simulink model "HighSpeedOperation"  (R2023a)
settings: Solver=VariableStepAuto  StartTime=0.0  StopTime=12  MaxStep=.00001  RelTol=.00001
values from neighbouring files (symbols this model uses):
  B = .005752    (= 0.005752)    [parameters.m]
  Fs = 5000    [parameters.m]
  I_rated = P_rated/(sqrt(3)*VLL_rms*.9*.9)    [parameters.m]
  J = .02    (= 0.02)    [parameters.m]
  lambda_r_rated = 0.94    [parameters.m]
  Llr = .005974    (= 0.005974)    [parameters.m]
  Lls = .005974    (= 0.005974)    [parameters.m]
  Lm = .2037    (= 0.2037)    [parameters.m]
  Lr = Lm+Llr    (= 0.209674)    [parameters.m]
  Ls = Lm+Lls    (= 0.209674)    [parameters.m]
  P = 4    [parameters.m]
  Rs = 1.115    [parameters.m]
  sigma = 1-((Lm)^2)/(Lr*Ls)    (= 0.0561719130296)    [parameters.m]
  Tr = Lr/Rr    (= 0.193604801477)    [parameters.m]
  Vdc = 600    [parameters.m]
  Vs_max = Vdc/sqrt(3)    [parameters.m]
libraries: slpidlib x7, spsMosfetLib x6, spsabctoAlphaBetaZeroLib x4, spsCurrentMeasurementLib x2, simulink x2, SignalEditorBlockLib x2, spsAsynchronousMachineSIUnitsLib x1, spsDCVoltageSourceLib x1, sps_lib x1
(part 1 of 2)
settings Model: Creator=User  LastModifiedBy=User
settings DebuggingCC: IgnoredZcDiagnostic=none

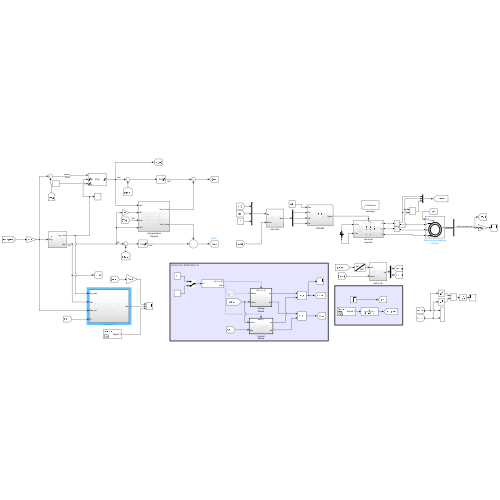
[thumbnail: Simulink's stored preview of the top-level diagram]
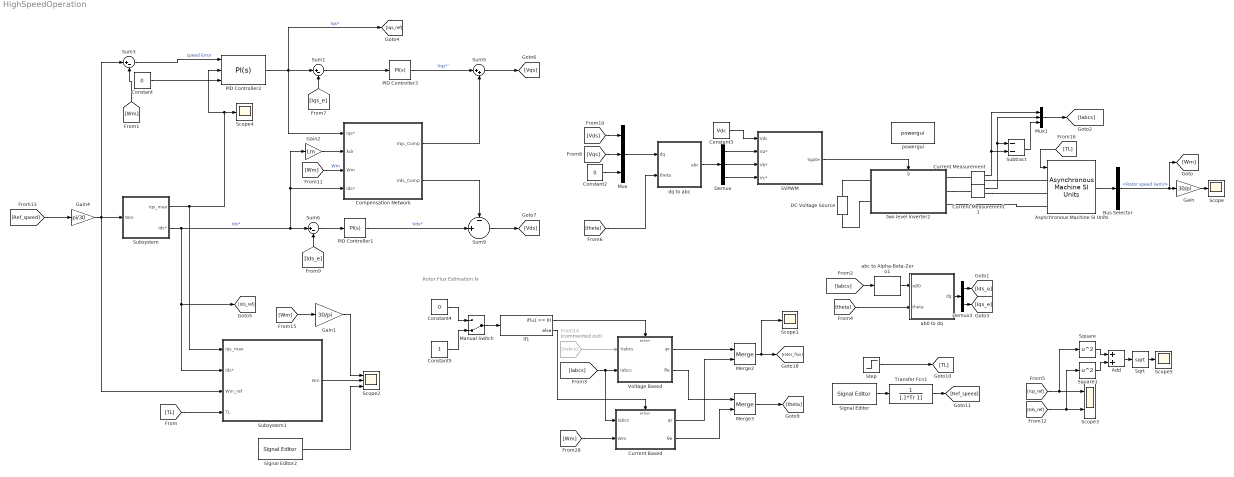
== system HighSpeedOperation ==
  note: Rotor Flux Estimation λr
  Add : Sum
  Asynchronous Machine SI Units : spsAsynchronousMachineSIUnitsLib/Asynchronous Machine SI Units  RotorType=Squirrel-cage  PresetModel="01:  5 HP   460 V 60Hz 1750 RPM"  MechanicalLoad=Torque Tm  ShowDetailedParameters=on  ReferenceFrame=Stationary  Units=SI  MeasurementBus=off  NominalParameters=[3730 460 60]  VoltageRatio=1  Stator=[1.115 0.005974]  Rotor=[1.083 0.005974]  Cage1=[0.4155 0.002066]  Cage2=[0.4168 0.0003495]  Lm=0.2037  Mechanical=[0.02 0.005752 2]  PolePairs=2  InitialConditions=[1 0 0 0 0 0 0 0]  SimulateSaturation=off  Saturation=[14.03593122, 27.81365428, 53.79336849, 72.68890987, 97.98006896, 148.6815601, 215.7428561, 302.9841135, 428.7778367 ; 230, 322, 414, 460, 506, 552, 598, 644, 690]  LoadFlowParameters=1492000  TsPowergui=0  TsBlock=-1  IterativeModel=Trapezoidal non iterative  IterativeDiscreteModel=Trapezoidal non iterative  Pmec=1.492e+006
  Bus Selector : BusSelector  OutputSignals=Mechanical.Rotor speed (wm)
  Compensation Network : Subsystem
  Constant : Constant  Value=0
  Constant2 : Constant  Value=0
  Constant3 : Constant  Value=Vdc
  Constant4 : Constant  Value=0
  Constant5 : Constant
  Current Based : Subsystem
  Current Measurement : spsCurrentMeasurementLib/Current Measurement  PhasorSimulation=off  OutputType=Complex  PSBequivalent=0
  Current Measurement1 : spsCurrentMeasurementLib/Current Measurement  PhasorSimulation=off  OutputType=Complex  PSBequivalent=0
  DC Voltage Source : spsDCVoltageSourceLib/DC Voltage Source  Amplitude=Vdc  Measurements=None
  Demux : Demux  Outputs=3
  Demux3 : Demux  Outputs=2
  From14 : From  Commented=on  GotoTag=Vabcs  TagVisibility=global
  Gain : Gain  Gain=30/pi
  Gain1 : Gain  Gain=30/pi
  Gain2 : Gain  Gain=Lm
  Gain4 : Gain  Gain=pi/30
  If1 : If  IfExpression=u1 == 0
  Manual Switch : ManualSwitch  CurrentSetting=0
  Merge2 : Merge
  Merge3 : Merge
  Mux : Mux  Inputs=3
  Mux1 : Mux  Inputs=3
  PID Controller1 : slpidlib/PID Controller  Controller=PI  Form=Parallel  TimeDomain=Continuous-time  UseExternalTs=off  SampleTime=-1  IntegratorMethod=Forward Euler  FilterMethod=Forward Euler  ControllerParametersSource=internal  P=8.96154169507065  I=1405.53236610577  UseKiTs=off  D=0  N=100  UseFilter=on  TunerSelectOption=Transfer Function Based (PID Tuner App)  InitialConditionSource=internal  InitialConditionForIntegrator=0  InitialConditionForFilter=0  DifferentiatorICPrevScaledInput=0  ExternalReset=none  TrackingMode=off  Kt=1  LimitOutput=on  SatLimitsSource=internal  UpperSaturationLimit=inf  LowerSaturationLimit=-inf  LinearizeAsGain=on  AntiWindupMode=clamping  Kb=1  LimitIntegrator=off  UpperIntegratorSaturationLimit=inf  LowerIntegratorSaturationLimit=-inf  POutMin=[]  POutMax=[]  IOutMin=[]  IOutMax=[]  DOutMin=[]  DOutMax=[]  NOutMin=[]  NOutMax=[]  SumOutMin=[]  SumOutMax=[]  SaturationOutMin=[]  SaturationOutMax=[]  PParamMin=[]  PParamMax=[]  IParamMin=[]  IParamMax=[]  DParamMin=[]  DParamMax=[]  NParamMin=[]  NParamMax=[]  KbParamMin=[]  KbParamMax=[]  KtParamMin=[]  KtParamMax=[]  KbOutMin=[]  KbOutMax=[]  KtOutMin=[]  KtOutMax=[]  IntegratorOutMin=[]  IntegratorOutMax=[]  FilterOutMin=[]  FilterOutMax=[]  SumI1OutMin=[]  SumI1OutMax=[]  SumI2OutMin=[]  SumI2OutMax=[]  SumI3OutMin=[]  SumI3OutMax=[]  SumI4OutMin=[]  SumI4OutMax=[]  SumDOutMin=[]  SumDOutMax=[]  DifferentiatorOutMin=[]  DifferentiatorOutMax=[]  FilterDiffOutCoefMin=[]  FilterDiffOutCoefMax=[]  ReciprocalOutMin=[]  ReciprocalOutMax=[]  SumDenOutMin=[]  SumDenOutMax=[]  SumNumOutMin=[]  SumNumOutMax=[]  DivideOutMin=[]  DivideOutMax=[]  UdiffTsProdOutMin=[]  UdiffTsProdOutMax=[]  NTsProdOutMin=[]  NTsProdOutMax=[]  UintegralTsProdOutMin=[]  UintegralTsProdOutMax=[]  UngainTsProdOutMin=[]  UngainTsProdOutMax=[]  ClampingZeroOutDataTypeStr=Inherit: Inherit via back propagation  ClampingZeroOutMin=[]  ClampingZeroOutMax=[]  FilterDenConstantOutDataTypeStr=Inherit: Inherit via back propagation  FilterDenConstantOutMin=[]  FilterDenConstantOutMax=[]  PCopyOutDataTypeStr=Inherit: Inherit via back propagation  PCopyOutMin=[]  PCopyOutMax=[]  NCopyOutDataTypeStr=Inherit: Inherit via back propagation  NCopyOutMin=[]  NCopyOutMax=[]  IntegratorContinuousStateAttributes=''  IntegratorStateMustResolveToSignalObject=off  IntegratorRTWStateStorageClass=Auto  FilterContinuousStateAttributes=''  FilterStateMustResolveToSignalObject=off  FilterRTWStateStorageClass=Auto  ParallelPVariant=InternalParameters  IdealPVariant=Disabled  IVariant=InternalParameters  DVariant=Disabled  IntegratorVariant=Continuous  SatVariant=Enabled  AWVariant=ContClampingParallel  PCopyVariant=Disabled  TRVariant=Disabled  FdbkBlocksVariant=Forward  IdealPFdbkVariant=Disabled  SatFdbkVariant=Disabled  DerivativeFilterVariant=Disabled  NVariant=Disabled  NCopyVariant=Disabled_SignalSpec  FilterICVariant=Disabled  IntegratorICVariant=InternalICs  ExternalResetVariant=Disabled  TRSumVariant=Passthrough  SumFdbkVariant=Disabled  SumVariant=Sum_PI  TsampFilterVariant=InternalTs  TsampNgainVariant=Passthrough  TsampIntegralVariant=Disabled_SignalSpec  ExternalSaturationOutDataTypeStr=Inherit: Same as second input
  PID Controller2 : slpidlib/PID Controller  Controller=PI  Form=Parallel  TimeDomain=Continuous-time  UseExternalTs=off  SampleTime=-1  IntegratorMethod=Forward Euler  FilterMethod=Forward Euler  ControllerParametersSource=internal  P=3.31333209954479  I=19.3873586247509  UseKiTs=off  D=0  N=100  UseFilter=on  TunerSelectOption=Transfer Function Based (PID Tuner App)  InitialConditionSource=internal  InitialConditionForIntegrator=0  InitialConditionForFilter=0  DifferentiatorICPrevScaledInput=0  ExternalReset=none  TrackingMode=off  Kt=1  LimitOutput=on  SatLimitsSource=external  UpperSaturationLimit=inf  LowerSaturationLimit=-inf  LinearizeAsGain=on  AntiWindupMode=clamping  Kb=1  LimitIntegrator=off  UpperIntegratorSaturationLimit=inf  LowerIntegratorSaturationLimit=-inf  POutMin=[]  POutMax=[]  IOutMin=[]  IOutMax=[]  DOutMin=[]  DOutMax=[]  NOutMin=[]  NOutMax=[]  SumOutMin=[]  SumOutMax=[]  SaturationOutMin=[]  SaturationOutMax=[]  PParamMin=[]  PParamMax=[]  IParamMin=[]  IParamMax=[]  DParamMin=[]  DParamMax=[]  NParamMin=[]  NParamMax=[]  KbParamMin=[]  KbParamMax=[]  KtParamMin=[]  KtParamMax=[]  KbOutMin=[]  KbOutMax=[]  KtOutMin=[]  KtOutMax=[]  IntegratorOutMin=[]  IntegratorOutMax=[]  FilterOutMin=[]  FilterOutMax=[]  SumI1OutMin=[]  SumI1OutMax=[]  SumI2OutMin=[]  SumI2OutMax=[]  SumI3OutMin=[]  SumI3OutMax=[]  SumI4OutMin=[]  SumI4OutMax=[]  SumDOutMin=[]  SumDOutMax=[]  DifferentiatorOutMin=[]  DifferentiatorOutMax=[]  FilterDiffOutCoefMin=[]  FilterDiffOutCoefMax=[]  ReciprocalOutMin=[]  ReciprocalOutMax=[]  SumDenOutMin=[]  SumDenOutMax=[]  SumNumOutMin=[]  SumNumOutMax=[]  DivideOutMin=[]  DivideOutMax=[]  UdiffTsProdOutMin=[]  UdiffTsProdOutMax=[]  NTsProdOutMin=[]  NTsProdOutMax=[]  UintegralTsProdOutMin=[]  UintegralTsProdOutMax=[]  UngainTsProdOutMin=[]  UngainTsProdOutMax=[]  ClampingZeroOutDataTypeStr=Inherit: Inherit via back propagation  ClampingZeroOutMin=[]  ClampingZeroOutMax=[]  FilterDenConstantOutDataTypeStr=Inherit: Inherit via back propagation  FilterDenConstantOutMin=[]  FilterDenConstantOutMax=[]  PCopyOutDataTypeStr=Inherit: Inherit via back propagation  PCopyOutMin=[]  PCopyOutMax=[]  NCopyOutDataTypeStr=Inherit: Inherit via back propagation  NCopyOutMin=[]  NCopyOutMax=[]  IntegratorContinuousStateAttributes=''  IntegratorStateMustResolveToSignalObject=off  IntegratorRTWStateStorageClass=Auto  FilterContinuousStateAttributes=''  FilterStateMustResolveToSignalObject=off  FilterRTWStateStorageClass=Auto  ParallelPVariant=InternalParameters  IdealPVariant=Disabled  IVariant=InternalParameters  DVariant=Disabled  IntegratorVariant=Continuous  SatVariant=External  AWVariant=ContClampingParallel  PCopyVariant=Disabled  TRVariant=Disabled  FdbkBlocksVariant=Forward  IdealPFdbkVariant=Disabled  SatFdbkVariant=Disabled  DerivativeFilterVariant=Disabled  NVariant=Disabled  NCopyVariant=Disabled_SignalSpec  FilterICVariant=Disabled  IntegratorICVariant=InternalICs  ExternalResetVariant=Disabled  TRSumVariant=Passthrough  SumFdbkVariant=Disabled  SumVariant=Sum_PI  TsampFilterVariant=InternalTs  TsampNgainVariant=Passthrough  TsampIntegralVariant=Disabled_SignalSpec  ExternalSaturationOutDataTypeStr=Inherit: Same as second input
  PID Controller3 : slpidlib/PID Controller  Controller=PI  Form=Parallel  TimeDomain=Continuous-time  UseExternalTs=off  SampleTime=-1  IntegratorMethod=Forward Euler  FilterMethod=Forward Euler  ControllerParametersSource=internal  P=8.96154169507065  I=1405.53236610577  UseKiTs=off  D=0  N=100  UseFilter=on  TunerSelectOption=Transfer Function Based (PID Tuner App)  InitialConditionSource=internal  InitialConditionForIntegrator=0  InitialConditionForFilter=0  DifferentiatorICPrevScaledInput=0  ExternalReset=none  TrackingMode=off  Kt=1  LimitOutput=on  SatLimitsSource=internal  UpperSaturationLimit=inf  LowerSaturationLimit=-inf  LinearizeAsGain=on  AntiWindupMode=clamping  Kb=1  LimitIntegrator=off  UpperIntegratorSaturationLimit=inf  LowerIntegratorSaturationLimit=-inf  POutMin=[]  POutMax=[]  IOutMin=[]  IOutMax=[]  DOutMin=[]  DOutMax=[]  NOutMin=[]  NOutMax=[]  SumOutMin=[]  SumOutMax=[]  SaturationOutMin=[]  SaturationOutMax=[]  PParamMin=[]  PParamMax=[]  IParamMin=[]  IParamMax=[]  DParamMin=[]  DParamMax=[]  NParamMin=[]  NParamMax=[]  KbParamMin=[]  KbParamMax=[]  KtParamMin=[]  KtParamMax=[]  KbOutMin=[]  KbOutMax=[]  KtOutMin=[]  KtOutMax=[]  IntegratorOutMin=[]  IntegratorOutMax=[]  FilterOutMin=[]  FilterOutMax=[]  SumI1OutMin=[]  SumI1OutMax=[]  SumI2OutMin=[]  SumI2OutMax=[]  SumI3OutMin=[]  SumI3OutMax=[]  SumI4OutMin=[]  SumI4OutMax=[]  SumDOutMin=[]  SumDOutMax=[]  DifferentiatorOutMin=[]  DifferentiatorOutMax=[]  FilterDiffOutCoefMin=[]  FilterDiffOutCoefMax=[]  ReciprocalOutMin=[]  ReciprocalOutMax=[]  SumDenOutMin=[]  SumDenOutMax=[]  SumNumOutMin=[]  SumNumOutMax=[]  DivideOutMin=[]  DivideOutMax=[]  UdiffTsProdOutMin=[]  UdiffTsProdOutMax=[]  NTsProdOutMin=[]  NTsProdOutMax=[]  UintegralTsProdOutMin=[]  UintegralTsProdOutMax=[]  UngainTsProdOutMin=[]  UngainTsProdOutMax=[]  ClampingZeroOutDataTypeStr=Inherit: Inherit via back propagation  ClampingZeroOutMin=[]  ClampingZeroOutMax=[]  FilterDenConstantOutDataTypeStr=Inherit: Inherit via back propagation  FilterDenConstantOutMin=[]  FilterDenConstantOutMax=[]  PCopyOutDataTypeStr=Inherit: Inherit via back propagation  PCopyOutMin=[]  PCopyOutMax=[]  NCopyOutDataTypeStr=Inherit: Inherit via back propagation  NCopyOutMin=[]  NCopyOutMax=[]  IntegratorContinuousStateAttributes=''  IntegratorStateMustResolveToSignalObject=off  IntegratorRTWStateStorageClass=Auto  FilterContinuousStateAttributes=''  FilterStateMustResolveToSignalObject=off  FilterRTWStateStorageClass=Auto  ParallelPVariant=InternalParameters  IdealPVariant=Disabled  IVariant=InternalParameters  DVariant=Disabled  IntegratorVariant=Continuous  SatVariant=Enabled  AWVariant=ContClampingParallel  PCopyVariant=Disabled  TRVariant=Disabled  FdbkBlocksVariant=Forward  IdealPFdbkVariant=Disabled  SatFdbkVariant=Disabled  DerivativeFilterVariant=Disabled  NVariant=Disabled  NCopyVariant=Disabled_SignalSpec  FilterICVariant=Disabled  IntegratorICVariant=InternalICs  ExternalResetVariant=Disabled  TRSumVariant=Passthrough  SumFdbkVariant=Disabled  SumVariant=Sum_PI  TsampFilterVariant=InternalTs  TsampNgainVariant=Passthrough  TsampIntegralVariant=Disabled_SignalSpec  ExternalSaturationOutDataTypeStr=Inherit: Same as second input
  SVPWM : Subsystem
  Scope{,1,4..5} (4 alike) : Scope
  Scope2 : Scope  NumInputPorts=3
  Scope3 : Scope  NumInputPorts=2
  Signal Editor : SignalEditorBlockLib/Signal Editor  FileName=speedRef.mat  ActiveScenario=Scenario  ActiveSignal=Signal 1  IsBus=off  OutputBusObjectStr=Bus: BusObject  SampleTime=0  Interpolate=off  ZeroCross=off  OutputAfterFinalValue=Setting to zero  Unit=inherit  PreserveSignalName=on  ApplySigPropsToAllScenarios=on
  Signal Editor2 : SignalEditorBlockLib/Signal Editor  FileName=speedRef.mat  ActiveScenario=Scenario  ActiveSignal=Signal 1  IsBus=off  OutputBusObjectStr=Bus: BusObject  SampleTime=0  Interpolate=off  ZeroCross=off  OutputAfterFinalValue=Setting to zero  Unit=inherit  PreserveSignalName=on  ApplySigPropsToAllScenarios=on
  Sqrt : Sqrt
  Square : Math  Operator=square
  Square1 : Math  Operator=square
  Step : Step  Time=0  After=5  SampleTime=0
  Subsystem : Subsystem
  Subsystem1 : Subsystem
  Subtract : Sum  Inputs=--
  Sum1 : Sum  Inputs=|+-
  Sum3 : Sum  Inputs=|+-
  Sum5 : Sum  Inputs=|++
  Sum6 : Sum  Inputs=|+-
  Sum9 : Sum  Inputs=-||+|||
  Transfer Fcn1 : TransferFcn  Denominator=[.1*Tr 1]
  Voltage Based : Subsystem
  ab0 to dq : Subsystem
  abc to Alpha-Beta-Zero1 : spsabctoAlphaBetaZeroLib/abc to Alpha-Beta-Zero
  dq to abc : Subsystem
  powergui : sps_lib/powergui  Priority=1  SimulationMode=Continuous  SampleTime=50e-6  frequency=60  Iterations=50  frequencyindice=60  Pbase=100e6  ErrMax=1e-4  UnitsV=kV  UnitsW=MW  buscounter=0  FunctionMessages=off  echomessages=off  EnableUseOfTLC=off  CurrentSourceSwitches=off  DisableSnubberDevices=off  DisableRonSwitches=off  DisableVfSwitches=off  DisplayEquations=off  AutomaticDiscreteSolvers=off  SolverType=Tustin/Backward Euler (TBE)  Interpol=off  ExternalGateDelay=off  methode=off  Ts=100  x0status=blocks  SPID=on  SwTol=0  HookPort=off  NonlinearTolerance=1e-4  nMaxIteration=100  ContinueOnMaxIteration=off  RestoreLinks=warning  ResistiveCurrentMeasurement=off  Frange=[0:2:500]  Ylog=off  Xlog=on  ShowGrid=off  save=off  variable=ZData  structure=0  ZoomFFT=off  StartTime=0.0  cycles=1  DisplayStyle=1  fundamental=60  FreqAxis=off  MaxFrequency=1000  frequencyindicesteady=1  RmsSteady=1  display=off
  two level inverter2 : Subsystem
      settings: PortSchema="{\"entries\":[{\"content\":{\"sides\":[{\"content\":{\"connectorIds\":[\"LConn1\",\"LConn2\"]},\"type\":\"ConnectorPlacement.EquallySpacedRectSide\",\"uuid\":\"55e8c7ab-b683-49a5-a161-880a4a34a0f9\"},{\"content\":{\"connectorIds\":[\"RConn1\",\"RConn2\",\"RConn3\"],\"side\":\"RIGHT\"},\"type\":\"ConnectorPlacement.EquallySpacedRectSide\",\"uuid\":\"1084cdad-92a7-4542-81ba-0d2d7dc45086\"},{\"content\":{\"connectorIds\":[\"In1\"],\"side\":\"TOP\"},\"type\":\"ConnectorPlacement.EquallySpacedRectSide\",\"uuid\":\"05644563-18ca-49ab-8dc2-f0892e459ff9\"}]},\"type\":\"ConnectorPlacement.EquallySpacedConnector\",\"uuid\":\"cbfd1c3e-716e-4f9c-8b43-b54633b99acd\"}],\"packageUris\":[\"http://schema.mathworks.com/mf0/Connector/R2020b\"],\"version\":\"1.0\"}"
  wires:
  Bus Selector/1 -> [Wm], Gain/1  "<Rotor speed (wm)>"
  Step/1 -> [TL]
  Gain/1 -> Scope/1
  Asynchronous Machine SI Units/1 -> Bus Selector/1
  [Iabcs] -> abc to Alpha-Beta-Zero1/1
  Sum3/1 -> PID Controller2/1  "speed Error"
  [Iqs_e] -> Sum1/2
  Sum1/1 -> PID Controller3/1
  PID Controller3/1 -> Sum5/1  "Vqs*`"
  Signal Editor/1 -> Transfer Fcn1/1
  Mux/1 -> dq to abc/1(dq)
  [Vqs] -> Mux/2
  Constant2/1 -> Mux/3
  Sum5/1 -> [Vqs]
  [Ids_e] -> Sum6/2
  PID Controller1/1 -> Sum9/2  "Vds*`"
  [Vds] -> Mux/1
  Sum9/1 -> [Vds]
  [TL] -> Asynchronous Machine SI Units/1
  [theta] -> dq to abc/2(theta)
  Sum6/1 -> PID Controller1/1
  Constant5/1 -> Manual Switch/2
  Manual Switch/1 -> If1/1
  Voltage Based/1(φr) -> Merge2/1
  From14/1 -> Voltage Based/1(Vabcs)
  [Wm] -> Current Based/2(Wm)
  Constant4/1 -> Manual Switch/1
  Current Based/2(θe) -> Merge3/2
  [Iabcs] -> Current Based/1(Iabcs), Voltage Based/2(Iabcs)
  Voltage Based/2(θe) -> Merge3/1
  Current Based/1(φr) -> Merge2/2
  Merge2/1 -> Scope1/1, [rotor_flux]
  If1/1 -> Voltage Based/Action
  If1/2 -> Current Based/Action
  Merge3/1 -> [theta]
  [Wm] -> Compensation Network/3(Wm)  "Wm"
  [Wm] -> Sum3/2
  [theta] -> ab0 to dq/2(theta)
  abc to Alpha-Beta-Zero1/1 -> ab0 to dq/1(αβ0)
  Demux3/1 -> [Ids_e]
  Demux3/2 -> [Iqs_e]
  ab0 to dq/1(dq) -> Demux3/1
  Compensation Network/1(Vqs_Comp) -> Sum5/2
  Compensation Network/2(Vds_Comp) -> Sum9/1
  Transfer Fcn1/1 -> [Ref_speed]
  Current Measurement/1 -> Mux1/1, Subtract/2
  Current Measurement1/1 -> Subtract/1, Mux1/2
  Mux1/1 -> [Iabcs]
  Subtract/1 -> Mux1/3
  Demux/1 -> SVPWM/2(Va*)
  Constant3/1 -> SVPWM/1(Vdc)
  Demux/2 -> SVPWM/3(Vb*)
  Demux/3 -> SVPWM/4(Vc*)
  dq to abc/1(abc) -> Demux/1
  SVPWM/1(Sgate) -> two level inverter2/1(g)
  [Iqs_ref] -> Scope3/1, Square/1
  [Ids_ref] -> Scope3/2, Square1/1
  [Ref_speed] -> Gain4/1
  Gain4/1 -> Subsystem1/3(Wm_ref), Sum3/1, Subsystem/1(Wm)
  [TL] -> Subsystem1/4(TL)
  PID Controller2/1 -> Compensation Network/1(Iqs*), Sum1/1, [Iqs_ref]  "Iqs*"
  Constant/1 -> PID Controller2/3
  [Wm] -> Gain1/1
  Subsystem1/1(Nm) -> Scope2/2
  Gain1/1 -> Scope2/1
  Signal Editor2/1 -> Scope2/3
  Subsystem/1(Iqs_max) -> Subsystem1/1(Iqs_max), PID Controller2/2, Scope4/1
  Gain2/1 -> Compensation Network/2(λdr)
  Subsystem/2(Ids*) -> [Ids_ref], Subsystem1/2(Ids*), Compensation Network/4(Ids*), Gain2/1, Sum6/1  "Ids*"
  Square/1 -> Add/1
  Square1/1 -> Add/2
  Add/1 -> Sqrt/1
  Sqrt/1 -> Scope5/1
  connections:
  two level inverter2/RConn1 -- Current Measurement/LConn1
  DC Voltage Source/LConn1 -- two level inverter2/LConn2
  DC Voltage Source/RConn1 -- two level inverter2/LConn1
  two level inverter2/RConn2 -- Current Measurement1/LConn1
  two level inverter2/RConn3 -- Asynchronous Machine SI Units/LConn3
  Current Measurement1/RConn1 -- Asynchronous Machine SI Units/LConn2
  Asynchronous Machine SI Units/LConn1 -- Current Measurement/RConn1

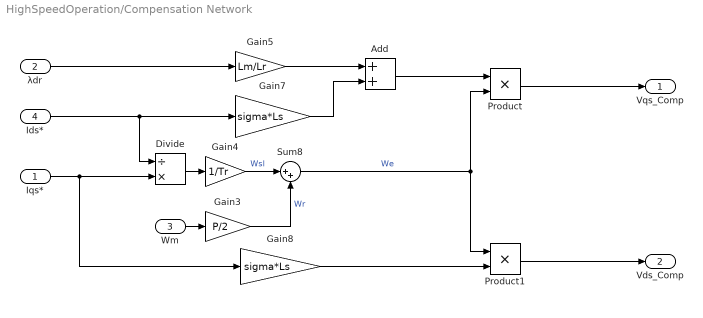
== system HighSpeedOperation/Compensation Network ==
  Iqs* : Inport
  λdr : Inport  Port=2
  Wm : Inport  Port=3
  Ids* : Inport  Port=4
  Add : Sum
  Divide : Product  Inputs=/*
  Gain3 : Gain  Gain=P/2
  Gain4 : Gain  Gain=1/Tr
  Gain5 : Gain  Gain=Lm/Lr
  Gain7 : Gain  Gain=sigma*Ls
  Gain8 : Gain  Gain=sigma*Ls
  Product : Product
  Product1 : Product
  Sum8 : Sum  Inputs=|++
  Vqs_Comp : Outport
  Vds_Comp : Outport  Port=2
  wires:
  Iqs*/1 -> Divide/2, Gain8/1
  Sum8/1 -> Product/2, Product1/1  "We"
  Product/1 -> Vqs_Comp/1
  Gain3/1 -> Sum8/2  "Wr"
  Ids*/1 -> Divide/1, Gain7/1
  Gain5/1 -> Add/1
  Gain7/1 -> Add/2
  Divide/1 -> Gain4/1
  λdr/1 -> Gain5/1
  Gain4/1 -> Sum8/1  "Wsl"
  Gain8/1 -> Product1/2
  Add/1 -> Product/1
  Wm/1 -> Gain3/1
  Product1/1 -> Vds_Comp/1

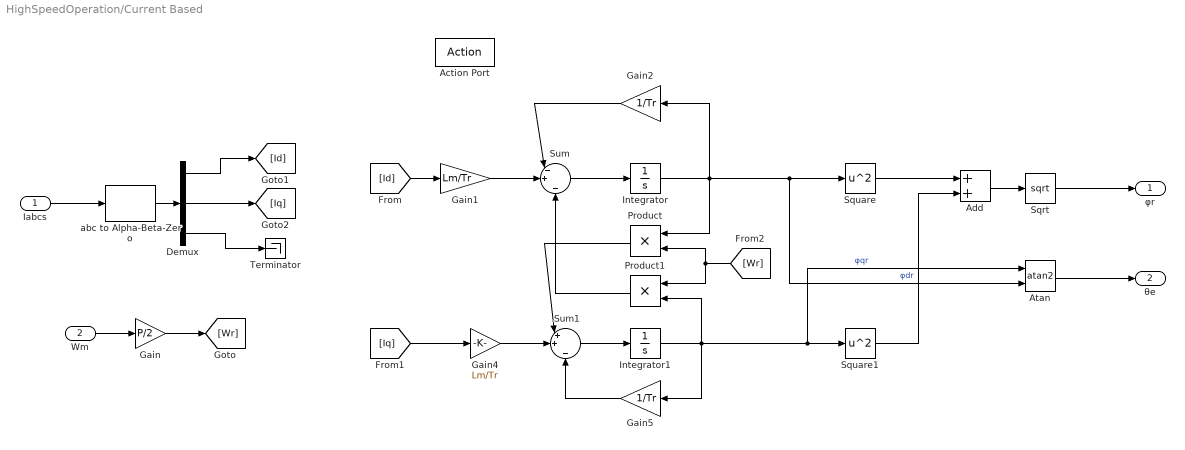
== system HighSpeedOperation/Current Based ==
  Iabcs : Inport
  Wm : Inport  Port=2
  Action Port : ActionPort  ActionPortLabel=else
  Add : Sum
  Atan : Trigonometry  Operator=atan2
  Demux : Demux  Outputs=3
  Gain : Gain  Gain=P/2
  Gain1 : Gain  Gain=Lm/Tr
  Gain2 : Gain  Gain=1/Tr
  Gain4 : Gain  Gain=Lm/Tr
  Gain5 : Gain  Gain=1/Tr
  Integrator : Integrator
  Integrator1 : Integrator
  Product : Product
  Product1 : Product
  Sqrt : Sqrt
  Square : Math  Operator=square
  Square1 : Math  Operator=square
  Sum : Sum  Inputs=|-+|-
  Sum1 : Sum  Inputs=|++|-
  Terminator : Terminator
  abc to Alpha-Beta-Zero : spsabctoAlphaBetaZeroLib/abc to Alpha-Beta-Zero
  φr : Outport
  θe : Outport  Port=2
  wires:
  Atan/1 -> θe/1
  Sqrt/1 -> φr/1
  Add/1 -> Sqrt/1
  Square1/1 -> Add/2
  Square/1 -> Add/1
  Gain5/1 -> Sum1/3
  Integrator/1 -> Product/1, Gain2/1, Atan/2, Square/1  "φdr"
  Product/1 -> Sum1/1
  Product1/1 -> Sum/3
  Integrator1/1 -> Product1/2, Atan/1, Square1/1, Gain5/1  "φqr"
  [Wr] -> Product1/1, Product/2
  [Iq] -> Gain4/1
  Gain4/1 -> Sum1/2
  Sum1/1 -> Integrator1/1
  Gain2/1 -> Sum/1
  Sum/1 -> Integrator/1
  Gain1/1 -> Sum/2
  [Id] -> Gain1/1
  Demux/3 -> Terminator/1
  Demux/2 -> [Iq]
  Demux/1 -> [Id]
  abc to Alpha-Beta-Zero/1 -> Demux/1
  Iabcs/1 -> abc to Alpha-Beta-Zero/1
  Gain/1 -> [Wr]
  Wm/1 -> Gain/1

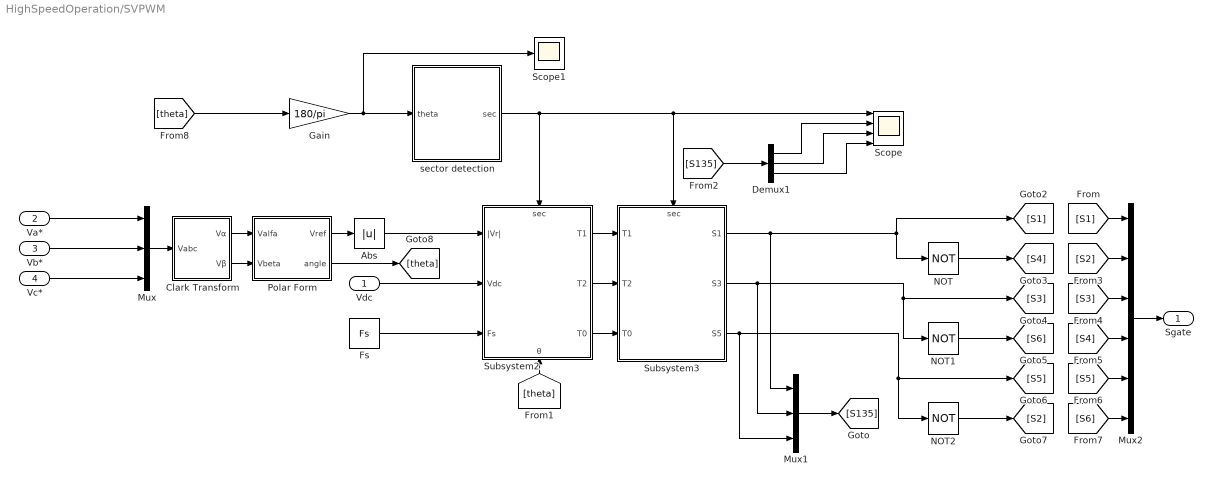
== system HighSpeedOperation/SVPWM ==
  Vdc : Inport
  Va* : Inport  Port=2
  Vb* : Inport  Port=3
  Vc* : Inport  Port=4
  Abs : Abs  SaturateOnIntegerOverflow=off
  "Clark Transform " : Subsystem
  Demux1 : Demux  Outputs=3
  Fs : Constant  Value=Fs
  Gain : Gain  Gain=180/pi
  Mux : Mux  Inputs=3
  Mux1 : Mux  Inputs=3
  Mux2 : Mux  Inputs=6
  NOT : Logic  Operator=NOT  IconShape=distinctive  AllPortsSameDT=off  OutDataTypeStr=boolean
  NOT1 : Logic  Operator=NOT  IconShape=distinctive  AllPortsSameDT=off  OutDataTypeStr=boolean
  NOT2 : Logic  Operator=NOT  IconShape=distinctive  AllPortsSameDT=off  OutDataTypeStr=boolean
  "Polar Form " : Subsystem
  Scope : Scope  NumInputPorts=4
  Scope1 : Scope
  Subsystem2 : Subsystem
      settings: PortSchema="{\"entries\":[{\"content\":{\"sides\":[{\"content\":{\"connectorIds\":[\"In1\",\"In2\",\"In3\"]},\"type\":\"ConnectorPlacement.EquallySpacedRectSide\",\"uuid\":\"13f95eee-8106-4f2d-b5f9-665b5c53ca49\"},{\"content\":{\"connectorIds\":[\"Out1\",\"Out2\",\"Out3\"],\"side\":\"RIGHT\"},\"type\":\"ConnectorPlacement.EquallySpacedRectSide\",\"uuid\":\"3e078310-26cc-4d9c-be70-8da9dd20e061\"},{\"content\":{\"connectorIds\":[\"In4\"],\"side\":\"TOP\"},\"type\":\"ConnectorPlacement.EquallySpacedRectSide\",\"uuid\":\"527b4023-fe6f-4401-b457-72fad21c543f\"},{\"content\":{\"connectorIds\":[\"In5\"],\"side\":\"BOTTOM\"},\"type\":\"ConnectorPlacement.EquallySpacedRectSide\",\"uuid\":\"69a9f471-00dd-451f-93ed-c0a69f4545a9\"}]},\"type\":\"ConnectorPlacement.EquallySpacedConnector\",\"uuid\":\"05647124-acf5-4dc1-bc20-aba6809c1c0b\"}],\"packageUris\":[\"http://schema.mathworks.com/mf0/Connector/R2020b\"],\"version\":\"1.0\"}"
  Subsystem3 : Subsystem
      settings: PortSchema="{\"entries\":[{\"content\":{\"sides\":[{\"content\":{\"connectorIds\":[\"In1\",\"In2\",\"In3\"]},\"type\":\"ConnectorPlacement.EquallySpacedRectSide\",\"uuid\":\"6c42d831-0426-4967-81f5-911cdfb3d9a5\"},{\"content\":{\"connectorIds\":[\"Out1\",\"Out2\",\"Out3\"],\"side\":\"RIGHT\"},\"type\":\"ConnectorPlacement.EquallySpacedRectSide\",\"uuid\":\"75f77ef2-8b2a-4026-a5e0-70e2e431df99\"},{\"content\":{\"connectorIds\":[\"In4\"],\"side\":\"TOP\"},\"type\":\"ConnectorPlacement.EquallySpacedRectSide\",\"uuid\":\"22b03ee4-555c-4834-b3ff-e7f6f70f60e9\"},{\"content\":{\"side\":\"BOTTOM\"},\"type\":\"ConnectorPlacement.EquallySpacedRectSide\",\"uuid\":\"5d3c1f0d-ee71-4b44-b9fa-21d524e176be\"}]},\"type\":\"ConnectorPlacement.EquallySpacedConnector\",\"uuid\":\"63507533-f8f6-475a-b41c-1823c26ae2e9\"}],\"packageUris\":[\"http://schema.mathworks.com/mf0/Connector/R2020b\"],\"version\":\"1.0\"}"
  sector detection : MATLAB Function  TreatAsAtomicUnit=on
  Sgate : Outport
  wires:
  Subsystem2/3(T0) -> Subsystem3/3(T0)
  Subsystem2/2(T2) -> Subsystem3/2(T2)
  Subsystem2/1(T1) -> Subsystem3/1(T1)
  Fs/1 -> Subsystem2/3(Fs)
  [theta] -> Subsystem2/5(" θ")
  sector detection/1(sec) -> Scope/1, Subsystem3/4(sec), Subsystem2/4(sec)
  "Polar Form "/1(Vref) -> Abs/1
  Mux/1 -> "Clark Transform "/1("Vabc ")
  NOT2/1 -> [S2]
  Subsystem3/3(S5) -> Mux1/3, [S5], NOT2/1
  Subsystem3/2(S3) -> Mux1/2, [S3], NOT1/1
  NOT/1 -> [S4]
  Subsystem3/1(S1) -> Mux1/1, [S1], NOT/1
  Vb*/1 -> Mux/2
  Vc*/1 -> Mux/3
  Vdc/1 -> Subsystem2/2(Vdc)
  Va*/1 -> Mux/1
  Mux1/1 -> [S135]
  [S135] -> Demux1/1
  Demux1/1 -> Scope/2
  Demux1/2 -> Scope/3
  Demux1/3 -> Scope/4
  Gain/1 -> Scope1/1, sector detection/1(theta)
  NOT1/1 -> [S6]
  Mux2/1 -> Sgate/1
  [S1] -> Mux2/1
  [S2] -> Mux2/2
  [S3] -> Mux2/3
  [S4] -> Mux2/4
  [S5] -> Mux2/5
  [S6] -> Mux2/6
  "Clark Transform "/1(Vα) -> "Polar Form "/1(Valfa)
  "Clark Transform "/2(Vβ) -> "Polar Form "/2(Vbeta)
  Abs/1 -> Subsystem2/1(|Vr|)
  [theta] -> Gain/1
  "Polar Form "/2(angle) -> [theta]

== system HighSpeedOperation/Subsystem ==
  Wm : Inport
  Constant Torque region : Subsystem  TreatAsAtomicUnit=on
  Field Weakening Region I : Subsystem  TreatAsAtomicUnit=on
  Field Weakening Region II : Subsystem  TreatAsAtomicUnit=on
  If : If  IfExpression=u1 < Wbase_FW_RegionI  ElseIfExpressions=Wbase_FW_RegionI < u1 < W_BT_RegionII
  Merge : Merge  Inputs=3
  Merge1 : Merge  Inputs=3
  Iqs_max : Outport
  Ids* : Outport  Port=2
  wires:
  Field Weakening Region I/1(Ids*) -> Merge/2
  Merge/1 -> Ids*/1
  If/1 -> Constant Torque region/Action
  If/2 -> Field Weakening Region I/Action
  Wm/1 -> Field Weakening Region I/1(Wm), Field Weakening Region II/1(Wm), If/1
  Constant Torque region/2(Iqs_max) -> Merge1/1
  Merge1/1 -> Iqs_max/1
  Field Weakening Region I/2(Iqs_max) -> Merge1/2
  If/3 -> Field Weakening Region II/Action
  Field Weakening Region II/1(Ids*) -> Merge/3
  Field Weakening Region II/2(Iqs_max) -> Merge1/3
  Constant Torque region/1(Ids*) -> Merge/1

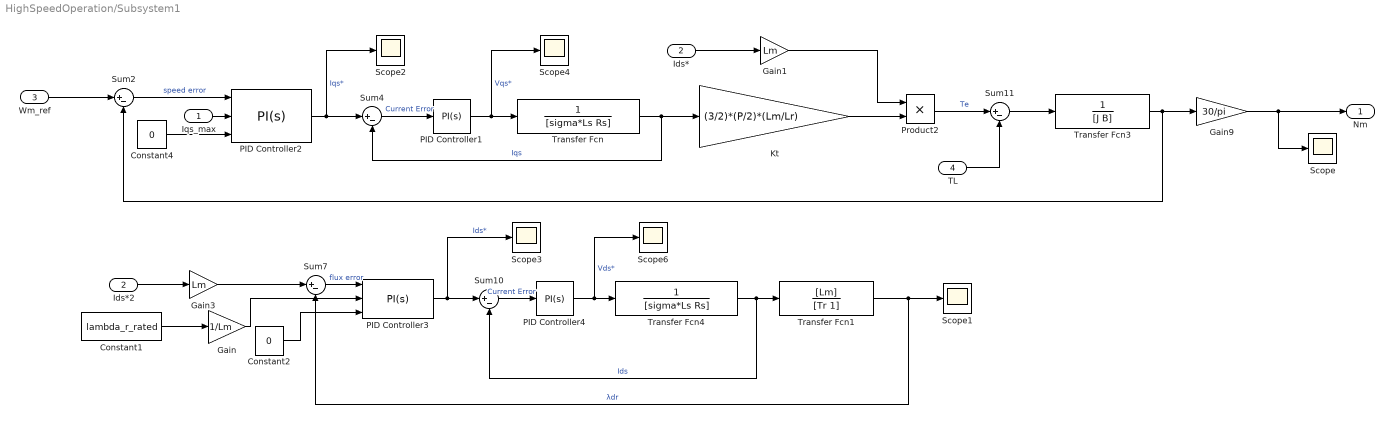
== system HighSpeedOperation/Subsystem1 ==
  Iqs_max : Inport
  Ids* : Inport  Port=2
  Wm_ref : Inport  Port=3
  TL : Inport  Port=4
  Constant1 : Constant  Value=lambda_r_rated
  Constant2 : Constant  Value=0
  Constant4 : Constant  Value=0
  Gain : Gain  Gain=1/Lm
  Gain1 : Gain  Gain=Lm
  Gain3 : Gain  Gain=Lm
  Gain9 : Gain  Gain=30/pi
  Ids*2 : InportShadow  Port=2
  Kt : Gain  Gain=(3/2)*(P/2)*(Lm/Lr)
  PID Controller1 : slpidlib/PID Controller  Controller=PI  Form=Parallel  TimeDomain=Continuous-time  UseExternalTs=off  SampleTime=-1  IntegratorMethod=Forward Euler  FilterMethod=Forward Euler  ControllerParametersSource=internal  P=8.96154169507065  I=1405.53236610577  UseKiTs=off  D=0  N=100  UseFilter=on  TunerSelectOption=Transfer Function Based (PID Tuner App)  InitialConditionSource=internal  InitialConditionForIntegrator=0  InitialConditionForFilter=0  DifferentiatorICPrevScaledInput=0  ExternalReset=none  TrackingMode=off  Kt=1  LimitOutput=on  SatLimitsSource=internal  UpperSaturationLimit=inf  LowerSaturationLimit=-inf  LinearizeAsGain=on  AntiWindupMode=clamping  Kb=1  LimitIntegrator=off  UpperIntegratorSaturationLimit=inf  LowerIntegratorSaturationLimit=-inf  POutMin=[]  POutMax=[]  IOutMin=[]  IOutMax=[]  DOutMin=[]  DOutMax=[]  NOutMin=[]  NOutMax=[]  SumOutMin=[]  SumOutMax=[]  SaturationOutMin=[]  SaturationOutMax=[]  PParamMin=[]  PParamMax=[]  IParamMin=[]  IParamMax=[]  DParamMin=[]  DParamMax=[]  NParamMin=[]  NParamMax=[]  KbParamMin=[]  KbParamMax=[]  KtParamMin=[]  KtParamMax=[]  KbOutMin=[]  KbOutMax=[]  KtOutMin=[]  KtOutMax=[]  IntegratorOutMin=[]  IntegratorOutMax=[]  FilterOutMin=[]  FilterOutMax=[]  SumI1OutMin=[]  SumI1OutMax=[]  SumI2OutMin=[]  SumI2OutMax=[]  SumI3OutMin=[]  SumI3OutMax=[]  SumI4OutMin=[]  SumI4OutMax=[]  SumDOutMin=[]  SumDOutMax=[]  DifferentiatorOutMin=[]  DifferentiatorOutMax=[]  FilterDiffOutCoefMin=[]  FilterDiffOutCoefMax=[]  ReciprocalOutMin=[]  ReciprocalOutMax=[]  SumDenOutMin=[]  SumDenOutMax=[]  SumNumOutMin=[]  SumNumOutMax=[]  DivideOutMin=[]  DivideOutMax=[]  UdiffTsProdOutMin=[]  UdiffTsProdOutMax=[]  NTsProdOutMin=[]  NTsProdOutMax=[]  UintegralTsProdOutMin=[]  UintegralTsProdOutMax=[]  UngainTsProdOutMin=[]  UngainTsProdOutMax=[]  ClampingZeroOutDataTypeStr=Inherit: Inherit via back propagation  ClampingZeroOutMin=[]  ClampingZeroOutMax=[]  FilterDenConstantOutDataTypeStr=Inherit: Inherit via back propagation  FilterDenConstantOutMin=[]  FilterDenConstantOutMax=[]  PCopyOutDataTypeStr=Inherit: Inherit via back propagation  PCopyOutMin=[]  PCopyOutMax=[]  NCopyOutDataTypeStr=Inherit: Inherit via back propagation  NCopyOutMin=[]  NCopyOutMax=[]  IntegratorContinuousStateAttributes=''  IntegratorStateMustResolveToSignalObject=off  IntegratorRTWStateStorageClass=Auto  FilterContinuousStateAttributes=''  FilterStateMustResolveToSignalObject=off  FilterRTWStateStorageClass=Auto  ParallelPVariant=InternalParameters  IdealPVariant=Disabled  IVariant=InternalParameters  DVariant=Disabled  IntegratorVariant=Continuous  SatVariant=Enabled  AWVariant=ContClampingParallel  PCopyVariant=Disabled  TRVariant=Disabled  FdbkBlocksVariant=Forward  IdealPFdbkVariant=Disabled  SatFdbkVariant=Disabled  DerivativeFilterVariant=Disabled  NVariant=Disabled  NCopyVariant=Disabled_SignalSpec  FilterICVariant=Disabled  IntegratorICVariant=InternalICs  ExternalResetVariant=Disabled  TRSumVariant=Passthrough  SumFdbkVariant=Disabled  SumVariant=Sum_PI  TsampFilterVariant=InternalTs  TsampNgainVariant=Passthrough  TsampIntegralVariant=Disabled_SignalSpec  ExternalSaturationOutDataTypeStr=Inherit: Same as second input
  PID Controller2 : slpidlib/PID Controller  Controller=PI  Form=Parallel  TimeDomain=Continuous-time  UseExternalTs=off  SampleTime=-1  IntegratorMethod=Forward Euler  FilterMethod=Forward Euler  ControllerParametersSource=internal  P=3.31333209954479  I=19.3873586247509  UseKiTs=off  D=0  N=100  UseFilter=on  TunerSelectOption=Transfer Function Based (PID Tuner App)  InitialConditionSource=internal  InitialConditionForIntegrator=0  InitialConditionForFilter=0  DifferentiatorICPrevScaledInput=0  ExternalReset=none  TrackingMode=off  Kt=1  LimitOutput=on  SatLimitsSource=external  UpperSaturationLimit=inf  LowerSaturationLimit=-inf  LinearizeAsGain=on  AntiWindupMode=clamping  Kb=1  LimitIntegrator=off  UpperIntegratorSaturationLimit=inf  LowerIntegratorSaturationLimit=-inf  POutMin=[]  POutMax=[]  IOutMin=[]  IOutMax=[]  DOutMin=[]  DOutMax=[]  NOutMin=[]  NOutMax=[]  SumOutMin=[]  SumOutMax=[]  SaturationOutMin=[]  SaturationOutMax=[]  PParamMin=[]  PParamMax=[]  IParamMin=[]  IParamMax=[]  DParamMin=[]  DParamMax=[]  NParamMin=[]  NParamMax=[]  KbParamMin=[]  KbParamMax=[]  KtParamMin=[]  KtParamMax=[]  KbOutMin=[]  KbOutMax=[]  KtOutMin=[]  KtOutMax=[]  IntegratorOutMin=[]  IntegratorOutMax=[]  FilterOutMin=[]  FilterOutMax=[]  SumI1OutMin=[]  SumI1OutMax=[]  SumI2OutMin=[]  SumI2OutMax=[]  SumI3OutMin=[]  SumI3OutMax=[]  SumI4OutMin=[]  SumI4OutMax=[]  SumDOutMin=[]  SumDOutMax=[]  DifferentiatorOutMin=[]  DifferentiatorOutMax=[]  FilterDiffOutCoefMin=[]  FilterDiffOutCoefMax=[]  ReciprocalOutMin=[]  ReciprocalOutMax=[]  SumDenOutMin=[]  SumDenOutMax=[]  SumNumOutMin=[]  SumNumOutMax=[]  DivideOutMin=[]  DivideOutMax=[]  UdiffTsProdOutMin=[]  UdiffTsProdOutMax=[]  NTsProdOutMin=[]  NTsProdOutMax=[]  UintegralTsProdOutMin=[]  UintegralTsProdOutMax=[]  UngainTsProdOutMin=[]  UngainTsProdOutMax=[]  ClampingZeroOutDataTypeStr=Inherit: Inherit via back propagation  ClampingZeroOutMin=[]  ClampingZeroOutMax=[]  FilterDenConstantOutDataTypeStr=Inherit: Inherit via back propagation  FilterDenConstantOutMin=[]  FilterDenConstantOutMax=[]  PCopyOutDataTypeStr=Inherit: Inherit via back propagation  PCopyOutMin=[]  PCopyOutMax=[]  NCopyOutDataTypeStr=Inherit: Inherit via back propagation  NCopyOutMin=[]  NCopyOutMax=[]  IntegratorContinuousStateAttributes=''  IntegratorStateMustResolveToSignalObject=off  IntegratorRTWStateStorageClass=Auto  FilterContinuousStateAttributes=''  FilterStateMustResolveToSignalObject=off  FilterRTWStateStorageClass=Auto  ParallelPVariant=InternalParameters  IdealPVariant=Disabled  IVariant=InternalParameters  DVariant=Disabled  IntegratorVariant=Continuous  SatVariant=External  AWVariant=ContClampingParallel  PCopyVariant=Disabled  TRVariant=Disabled  FdbkBlocksVariant=Forward  IdealPFdbkVariant=Disabled  SatFdbkVariant=Disabled  DerivativeFilterVariant=Disabled  NVariant=Disabled  NCopyVariant=Disabled_SignalSpec  FilterICVariant=Disabled  IntegratorICVariant=InternalICs  ExternalResetVariant=Disabled  TRSumVariant=Passthrough  SumFdbkVariant=Disabled  SumVariant=Sum_PI  TsampFilterVariant=InternalTs  TsampNgainVariant=Passthrough  TsampIntegralVariant=Disabled_SignalSpec  ExternalSaturationOutDataTypeStr=Inherit: Same as second input
  PID Controller3 : slpidlib/PID Controller  Controller=PI  Form=Parallel  TimeDomain=Continuous-time  UseExternalTs=off  SampleTime=-1  IntegratorMethod=Forward Euler  FilterMethod=Forward Euler  ControllerParametersSource=internal  P=263.675956035498  I=1286.90873450599  UseKiTs=off  D=0  N=100  UseFilter=on  TunerSelectOption=Transfer Function Based (PID Tuner App)  InitialConditionSource=internal  InitialConditionForIntegrator=0  InitialConditionForFilter=0  DifferentiatorICPrevScaledInput=0  ExternalReset=none  TrackingMode=off  Kt=1  LimitOutput=on  SatLimitsSource=external  UpperSaturationLimit=inf  LowerSaturationLimit=-inf  LinearizeAsGain=on  AntiWindupMode=clamping  Kb=1  LimitIntegrator=off  UpperIntegratorSaturationLimit=inf  LowerIntegratorSaturationLimit=-inf  POutMin=[]  POutMax=[]  IOutMin=[]  IOutMax=[]  DOutMin=[]  DOutMax=[]  NOutMin=[]  NOutMax=[]  SumOutMin=[]  SumOutMax=[]  SaturationOutMin=[]  SaturationOutMax=[]  PParamMin=[]  PParamMax=[]  IParamMin=[]  IParamMax=[]  DParamMin=[]  DParamMax=[]  NParamMin=[]  NParamMax=[]  KbParamMin=[]  KbParamMax=[]  KtParamMin=[]  KtParamMax=[]  KbOutMin=[]  KbOutMax=[]  KtOutMin=[]  KtOutMax=[]  IntegratorOutMin=[]  IntegratorOutMax=[]  FilterOutMin=[]  FilterOutMax=[]  SumI1OutMin=[]  SumI1OutMax=[]  SumI2OutMin=[]  SumI2OutMax=[]  SumI3OutMin=[]  SumI3OutMax=[]  SumI4OutMin=[]  SumI4OutMax=[]  SumDOutMin=[]  SumDOutMax=[]  DifferentiatorOutMin=[]  DifferentiatorOutMax=[]  FilterDiffOutCoefMin=[]  FilterDiffOutCoefMax=[]  ReciprocalOutMin=[]  ReciprocalOutMax=[]  SumDenOutMin=[]  SumDenOutMax=[]  SumNumOutMin=[]  SumNumOutMax=[]  DivideOutMin=[]  DivideOutMax=[]  UdiffTsProdOutMin=[]  UdiffTsProdOutMax=[]  NTsProdOutMin=[]  NTsProdOutMax=[]  UintegralTsProdOutMin=[]  UintegralTsProdOutMax=[]  UngainTsProdOutMin=[]  UngainTsProdOutMax=[]  ClampingZeroOutDataTypeStr=Inherit: Inherit via back propagation  ClampingZeroOutMin=[]  ClampingZeroOutMax=[]  FilterDenConstantOutDataTypeStr=Inherit: Inherit via back propagation  FilterDenConstantOutMin=[]  FilterDenConstantOutMax=[]  PCopyOutDataTypeStr=Inherit: Inherit via back propagation  PCopyOutMin=[]  PCopyOutMax=[]  NCopyOutDataTypeStr=Inherit: Inherit via back propagation  NCopyOutMin=[]  NCopyOutMax=[]  IntegratorContinuousStateAttributes=''  IntegratorStateMustResolveToSignalObject=off  IntegratorRTWStateStorageClass=Auto  FilterContinuousStateAttributes=''  FilterStateMustResolveToSignalObject=off  FilterRTWStateStorageClass=Auto  ParallelPVariant=InternalParameters  IdealPVariant=Disabled  IVariant=InternalParameters  DVariant=Disabled  IntegratorVariant=Continuous  SatVariant=External  AWVariant=ContClampingParallel  PCopyVariant=Disabled  TRVariant=Disabled  FdbkBlocksVariant=Forward  IdealPFdbkVariant=Disabled  SatFdbkVariant=Disabled  DerivativeFilterVariant=Disabled  NVariant=Disabled  NCopyVariant=Disabled_SignalSpec  FilterICVariant=Disabled  IntegratorICVariant=InternalICs  ExternalResetVariant=Disabled  TRSumVariant=Passthrough  SumFdbkVariant=Disabled  SumVariant=Sum_PI  TsampFilterVariant=InternalTs  TsampNgainVariant=Passthrough  TsampIntegralVariant=Disabled_SignalSpec  ExternalSaturationOutDataTypeStr=Inherit: Same as second input
  PID Controller4 : slpidlib/PID Controller  Controller=PI  Form=Parallel  TimeDomain=Continuous-time  UseExternalTs=off  SampleTime=-1  IntegratorMethod=Forward Euler  FilterMethod=Forward Euler  ControllerParametersSource=internal  P=8.96154169507065  I=1405.53236610577  UseKiTs=off  D=0  N=100  UseFilter=on  TunerSelectOption=Transfer Function Based (PID Tuner App)  InitialConditionSource=internal  InitialConditionForIntegrator=0  InitialConditionForFilter=0  DifferentiatorICPrevScaledInput=0  ExternalReset=none  TrackingMode=off  Kt=1  LimitOutput=on  SatLimitsSource=internal  UpperSaturationLimit=inf  LowerSaturationLimit=-inf  LinearizeAsGain=on  AntiWindupMode=clamping  Kb=1  LimitIntegrator=off  UpperIntegratorSaturationLimit=inf  LowerIntegratorSaturationLimit=-inf  POutMin=[]  POutMax=[]  IOutMin=[]  IOutMax=[]  DOutMin=[]  DOutMax=[]  NOutMin=[]  NOutMax=[]  SumOutMin=[]  SumOutMax=[]  SaturationOutMin=[]  SaturationOutMax=[]  PParamMin=[]  PParamMax=[]  IParamMin=[]  IParamMax=[]  DParamMin=[]  DParamMax=[]  NParamMin=[]  NParamMax=[]  KbParamMin=[]  KbParamMax=[]  KtParamMin=[]  KtParamMax=[]  KbOutMin=[]  KbOutMax=[]  KtOutMin=[]  KtOutMax=[]  IntegratorOutMin=[]  IntegratorOutMax=[]  FilterOutMin=[]  FilterOutMax=[]  SumI1OutMin=[]  SumI1OutMax=[]  SumI2OutMin=[]  SumI2OutMax=[]  SumI3OutMin=[]  SumI3OutMax=[]  SumI4OutMin=[]  SumI4OutMax=[]  SumDOutMin=[]  SumDOutMax=[]  DifferentiatorOutMin=[]  DifferentiatorOutMax=[]  FilterDiffOutCoefMin=[]  FilterDiffOutCoefMax=[]  ReciprocalOutMin=[]  ReciprocalOutMax=[]  SumDenOutMin=[]  SumDenOutMax=[]  SumNumOutMin=[]  SumNumOutMax=[]  DivideOutMin=[]  DivideOutMax=[]  UdiffTsProdOutMin=[]  UdiffTsProdOutMax=[]  NTsProdOutMin=[]  NTsProdOutMax=[]  UintegralTsProdOutMin=[]  UintegralTsProdOutMax=[]  UngainTsProdOutMin=[]  UngainTsProdOutMax=[]  ClampingZeroOutDataTypeStr=Inherit: Inherit via back propagation  ClampingZeroOutMin=[]  ClampingZeroOutMax=[]  FilterDenConstantOutDataTypeStr=Inherit: Inherit via back propagation  FilterDenConstantOutMin=[]  FilterDenConstantOutMax=[]  PCopyOutDataTypeStr=Inherit: Inherit via back propagation  PCopyOutMin=[]  PCopyOutMax=[]  NCopyOutDataTypeStr=Inherit: Inherit via back propagation  NCopyOutMin=[]  NCopyOutMax=[]  IntegratorContinuousStateAttributes=''  IntegratorStateMustResolveToSignalObject=off  IntegratorRTWStateStorageClass=Auto  FilterContinuousStateAttributes=''  FilterStateMustResolveToSignalObject=off  FilterRTWStateStorageClass=Auto  ParallelPVariant=InternalParameters  IdealPVariant=Disabled  IVariant=InternalParameters  DVariant=Disabled  IntegratorVariant=Continuous  SatVariant=Enabled  AWVariant=ContClampingParallel  PCopyVariant=Disabled  TRVariant=Disabled  FdbkBlocksVariant=Forward  IdealPFdbkVariant=Disabled  SatFdbkVariant=Disabled  DerivativeFilterVariant=Disabled  NVariant=Disabled  NCopyVariant=Disabled_SignalSpec  FilterICVariant=Disabled  IntegratorICVariant=InternalICs  ExternalResetVariant=Disabled  TRSumVariant=Passthrough  SumFdbkVariant=Disabled  SumVariant=Sum_PI  TsampFilterVariant=InternalTs  TsampNgainVariant=Passthrough  TsampIntegralVariant=Disabled_SignalSpec  ExternalSaturationOutDataTypeStr=Inherit: Same as second input
  Product2 : Product
  Scope{,1..4,6} (6 alike) : Scope
  Sum{2,4,7,10..11} (5 alike) : Sum  Inputs=|+-
  Transfer Fcn : TransferFcn  Denominator=[sigma*Ls Rs]
  Transfer Fcn1 : TransferFcn  Numerator=[Lm]  Denominator=[Tr 1]
  Transfer Fcn3 : TransferFcn  Denominator=[J B]
  Transfer Fcn4 : TransferFcn  Denominator=[sigma*Ls Rs]
  Nm : Outport
  wires:
  PID Controller2/1 -> Scope2/1, Sum4/1  "Iqs*"
  Gain3/1 -> Sum7/1
  Sum2/1 -> PID Controller2/1  "speed error"
  PID Controller3/1 -> Sum10/1, Scope3/1  "Ids*"
  Sum7/1 -> PID Controller3/1  "flux error"
  Kt/1 -> Product2/2
  Gain9/1 -> Nm/1, Scope/1
  Transfer Fcn/1 -> Kt/1, Sum4/2  "Iqs"
  PID Controller1/1 -> Scope4/1, Transfer Fcn/1  "Vqs*"
  Transfer Fcn3/1 -> Sum2/2, Gain9/1
  Sum4/1 -> PID Controller1/1  "Current Error"
  Product2/1 -> Sum11/1  "Te"
  Sum10/1 -> PID Controller4/1  "Current Error"
  Transfer Fcn4/1 -> Transfer Fcn1/1, Sum10/2  "Ids"
  Gain1/1 -> Product2/1
  PID Controller4/1 -> Scope6/1, Transfer Fcn4/1  "Vds*"
  Sum11/1 -> Transfer Fcn3/1
  Wm_ref/1 -> Sum2/1
  TL/1 -> Sum11/2
  Constant4/1 -> PID Controller2/3
  Gain/1 -> PID Controller3/2
  Constant2/1 -> PID Controller3/3
  Transfer Fcn1/1 -> Scope1/1, Sum7/2  "λdr"
  Ids*/1 -> Gain1/1
  Ids*2/1 -> Gain3/1
  Constant1/1 -> Gain/1
  Iqs_max/1 -> PID Controller2/2

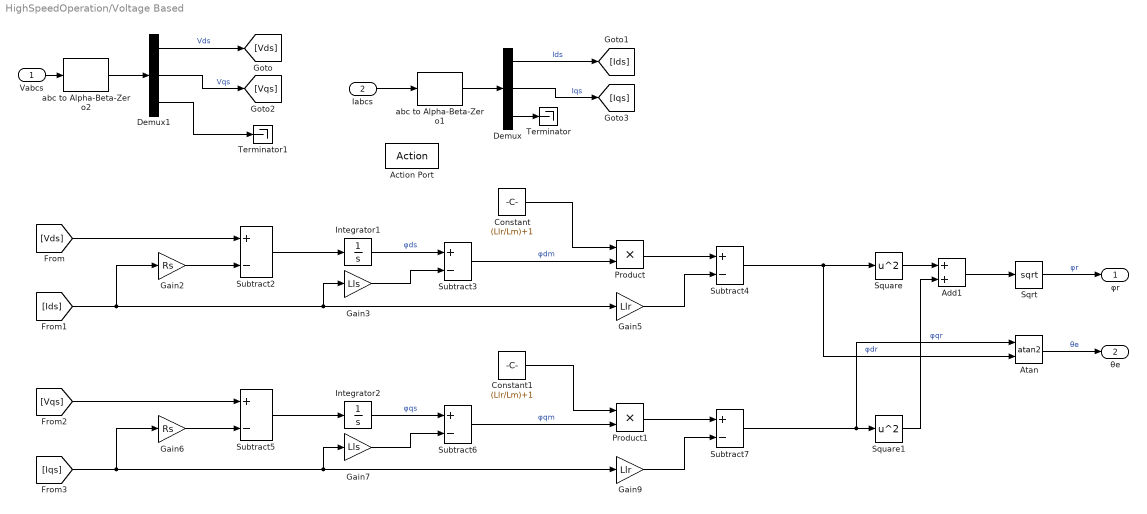
== system HighSpeedOperation/Voltage Based ==
  Vabcs : Inport
  Iabcs : Inport  Port=2
  Action Port : ActionPort  ActionPortLabel=if(u1 == 0)
  Add1 : Sum
  Atan : Trigonometry  Operator=atan2
  Constant : Constant  Value=(Llr/Lm)+1
  Constant1 : Constant  Value=(Llr/Lm)+1
  Demux : Demux  Outputs=3
  Demux1 : Demux  Outputs=3
  Gain2 : Gain  Gain=Rs
  Gain3 : Gain  Gain=Lls
  Gain5 : Gain  Gain=Llr
  Gain6 : Gain  Gain=Rs
  Gain7 : Gain  Gain=Lls
  Gain9 : Gain  Gain=Llr
  Integrator1 : Integrator
  Integrator2 : Integrator
  Product : Product
  Product1 : Product
  Sqrt : Sqrt
  Square : Math  Operator=square
  Square1 : Math  Operator=square
  Subtract{2..7} (6 alike) : Sum  Inputs=+-
  Terminator : Terminator
  Terminator1 : Terminator
  abc to Alpha-Beta-Zero1 : spsabctoAlphaBetaZeroLib/abc to Alpha-Beta-Zero
  abc to Alpha-Beta-Zero2 : spsabctoAlphaBetaZeroLib/abc to Alpha-Beta-Zero
  φr : Outport
  θe : Outport  Port=2
  wires:
  Iabcs/1 -> abc to Alpha-Beta-Zero1/1
  abc to Alpha-Beta-Zero1/1 -> Demux/1
  Demux/1 -> [Ids]  "Ids"
  Demux/2 -> [Iqs]  "Iqs"
  Demux1/2 -> [Vqs]  "Vqs"
  Demux1/1 -> [Vds]  "Vds"
  Demux/3 -> Terminator/1
  [Vds] -> Subtract2/1
  Gain2/1 -> Subtract2/2
  [Ids] -> Gain3/1, Gain5/1, Gain2/1
  Subtract2/1 -> Integrator1/1
  Integrator1/1 -> Subtract3/1  "φds"
  Gain3/1 -> Subtract3/2
  Subtract3/1 -> Product/2  "φdm"
  Constant/1 -> Product/1
  Product/1 -> Subtract4/1
  Gain5/1 -> Subtract4/2
  Subtract4/1 -> Atan/2, Square/1  "φdr"
  Subtract7/1 -> Atan/1, Square1/1  "φqr"
  Gain9/1 -> Subtract7/2
  Product1/1 -> Subtract7/1
  Subtract6/1 -> Product1/2  "φqm"
  Gain7/1 -> Subtract6/2
  Integrator2/1 -> Subtract6/1  "φqs"
  Subtract5/1 -> Integrator2/1
  [Iqs] -> Gain6/1, Gain9/1, Gain7/1
  Gain6/1 -> Subtract5/2
  [Vqs] -> Subtract5/1
  Square/1 -> Add1/1
  Add1/1 -> Sqrt/1
  Square1/1 -> Add1/2
  Sqrt/1 -> φr/1  "φr"
  Atan/1 -> θe/1  "θe"
  Constant1/1 -> Product1/1
  Vabcs/1 -> abc to Alpha-Beta-Zero2/1
  Demux1/3 -> Terminator1/1
  abc to Alpha-Beta-Zero2/1 -> Demux1/1

== system HighSpeedOperation/ab0 to dq ==
  αβ0 : Inport
  theta : Inport  Port=2
  Demux : Demux  Outputs=3
  Fcn : Fcn  Expr=u(1)*cos(u(4))+u(2)*sin(u(4))
  Fcn1 : Fcn  Expr=-u(1)*sin(u(4))+u(2)*cos(u(4))
  Mux : Mux
  Mux1 : Mux  Inputs=2
  dq : Outport
  wires:
  Mux/1 -> Fcn/1, Fcn1/1
  Fcn/1 -> Mux1/1  "d-axis"
  αβ0/1 -> Demux/1
  Demux/1 -> Mux/1  "alpha-axis"
  Demux/3 -> Mux/3  "0-axis"
  Demux/2 -> Mux/2  "beta-axis"
  theta/1 -> Mux/4  "theta"
  Fcn1/1 -> Mux1/2  "q-axis"
  Mux1/1 -> dq/1

== system HighSpeedOperation/dq to abc ==
  dq : Inport
  theta : Inport  Port=2
  Demux : Demux  Outputs=3
  Fcn : Fcn  Expr=u(1)*cos(u(4))-u(2)*sin(u(4))+u(3)
  Fcn1 : Fcn  Expr=u(1)*cos(u(4)-(2*pi/3))-u(2)*sin(u(4)-(2*pi/3))+u(3)
  Fcn3 : Fcn  Expr=u(1)*cos(u(4)+(2*pi/3))-u(2)*sin(u(4)+(2*pi/3))+u(3)
  Mux : Mux
  Mux1 : Mux  Inputs=3
  abc : Outport
  wires:
  Fcn/1 -> Mux1/1  "a-axis"
  Fcn3/1 -> Mux1/3  "c-axis"
  dq/1 -> Demux/1
  Demux/1 -> Mux/1  "d-axis"
  Demux/3 -> Mux/3  "0-axis"
  Demux/2 -> Mux/2  "q-axis"
  theta/1 -> Mux/4  "theta"
  Mux/1 -> Fcn3/1, Fcn1/1, Fcn/1
  Fcn1/1 -> Mux1/2  "b-axis"
  Mux1/1 -> abc/1

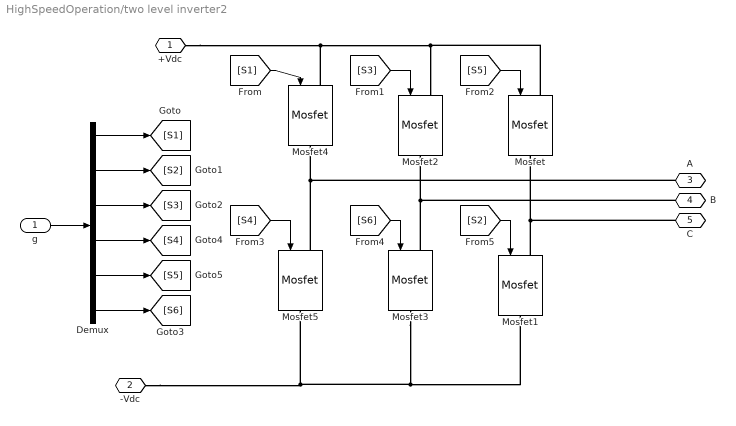
== system HighSpeedOperation/two level inverter2 ==
  g : Inport
  Demux : Demux  Outputs=6
  Mosfet{,1..5} (6 alike) : spsMosfetLib/Mosfet  Ron=0.1  Lon=0  Rd=0.01  Vfd=0  IC=0  Rs=1e5  Cs=inf  Measurements=off
  +Vdc : PMIOPort  Side=Left
  -Vdc : PMIOPort  Port=2  Side=Left
  A : PMIOPort  Port=3  Side=Right
  B : PMIOPort  Port=4  Side=Right
  C : PMIOPort  Port=5  Side=Right
  wires:
  g/1 -> Demux/1
  Demux/1 -> [S1]
  Demux/2 -> [S2]
  Demux/3 -> [S3]
  Demux/4 -> [S4]
  Demux/5 -> [S5]
  Demux/6 -> [S6]
  [S1] -> Mosfet4/1
  [S3] -> Mosfet2/1
  [S5] -> Mosfet/1
  [S4] -> Mosfet5/1
  [S6] -> Mosfet3/1
  [S2] -> Mosfet1/1
  connections:
  Mosfet4/LConn1 -- +Vdc/RConn1 -- Mosfet/LConn1 -- Mosfet2/LConn1
  Mosfet3/RConn1 -- Mosfet1/RConn1 -- -Vdc/RConn1 -- Mosfet5/RConn1
  Mosfet1/LConn1 -- Mosfet/RConn1 -- C/RConn1
  Mosfet3/LConn1 -- B/RConn1 -- Mosfet2/RConn1
  A/RConn1 -- Mosfet5/LConn1 -- Mosfet4/RConn1

== system HighSpeedOperation/SVPWM/Clark Transform  ==
  "Vabc " : Inport
  Fcn : Fcn  Expr=(u(1)-1/2*u(2)-1/2*u(3))
  Fcn1 : Fcn  Expr=(0*u(1)+sqrt(3)/2*u(2)-sqrt(3)/2*u(3))
  Vα : Outport  VectorParamsAs1DForOutWhenUnconnected=off
  Vβ : Outport  Port=2  VectorParamsAs1DForOutWhenUnconnected=off
  wires:
  Fcn/1 -> Vα/1
  "Vabc "/1 -> Fcn1/1, Fcn/1
  Fcn1/1 -> Vβ/1

== system HighSpeedOperation/SVPWM/Polar Form  ==
  Valfa : Inport
  Vbeta : Inport  Port=2
  Add : Sum
  Constant : Constant  Value=2*pi
  Fcn2 : Fcn  Expr=atan2(u(2),u(1))
  Fcn3 : Fcn  Expr=sqrt(u(1)^2+u(2)^2)
  Mux1 : Mux  Inputs=2
  Switch : Switch  Criteria=u2 > Threshold  SaturateOnIntegerOverflow=off  InputSameDT=off
  Vref : Outport  VectorParamsAs1DForOutWhenUnconnected=off
  angle : Outport  Port=2  VectorParamsAs1DForOutWhenUnconnected=off
  wires:
  Mux1/1 -> Fcn2/1, Fcn3/1
  Fcn3/1 -> Vref/1
  Valfa/1 -> Mux1/1
  Vbeta/1 -> Mux1/2
  Fcn2/1 -> Add/1, Switch/1, Switch/2
  Switch/1 -> angle/1
  Add/1 -> Switch/3
  Constant/1 -> Add/2

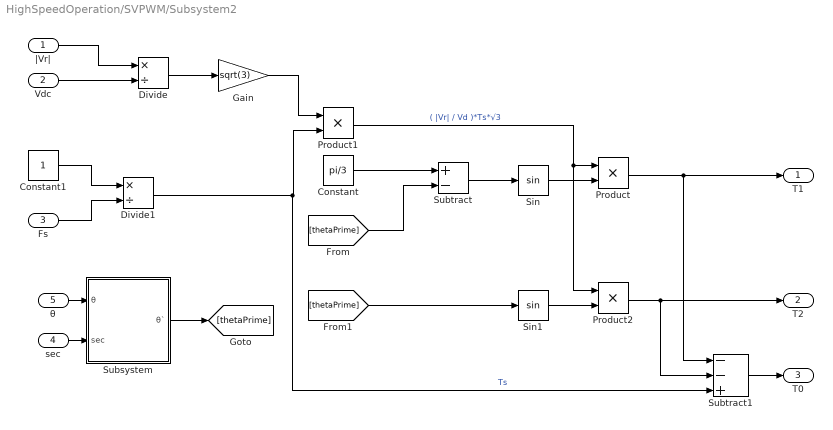
== system HighSpeedOperation/SVPWM/Subsystem2 ==
  |Vr| : Inport
  Vdc : Inport  Port=2
  Fs : Inport  Port=3
  sec : Inport  Port=4
  " θ" : Inport  Port=5
  Constant : Constant  Value=pi/3
  Constant1 : Constant
  Divide : Product  Inputs=*/
  Divide1 : Product  Inputs=*/
  Gain : Gain  Gain=sqrt(3)
  Product : Product
  Product1 : Product
  Product2 : Product
  Sin : Trigonometry
  Sin1 : Trigonometry
  Subsystem : Subsystem
  Subtract : Sum  Inputs=+-
  Subtract1 : Sum  Inputs=--+
  T1 : Outport
  T2 : Outport  Port=2
  T0 : Outport  Port=3
  wires:
  Subtract1/1 -> T0/1
  [thetaPrime] -> Sin1/1
  Sin1/1 -> Product2/2
  Product2/1 -> T2/1, Subtract1/2
  Gain/1 -> Product1/1
  Divide1/1 -> Product1/2, Subtract1/3  "Ts"
  Constant1/1 -> Divide1/1
  Fs/1 -> Divide1/2
  Divide/1 -> Gain/1
  Product1/1 -> Product/1, Product2/1  "( |Vr| / Vd )*Ts*√3"
  Vdc/1 -> Divide/2
  |Vr|/1 -> Divide/1
  Product/1 -> T1/1, Subtract1/1
  Sin/1 -> Product/2
  Subtract/1 -> Sin/1
  [thetaPrime] -> Subtract/2
  Subsystem/1(θ`) -> [thetaPrime]
  sec/1 -> Subsystem/2(sec)
  Constant/1 -> Subtract/1
  " θ"/1 -> Subsystem/1(θ)

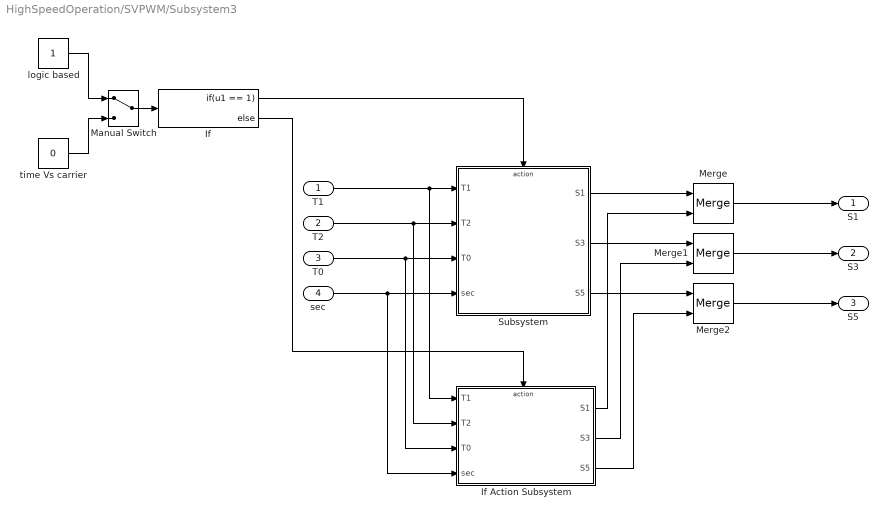
== system HighSpeedOperation/SVPWM/Subsystem3 ==
  T1 : Inport
  T2 : Inport  Port=2
  T0 : Inport  Port=3
  sec : Inport  Port=4
  If : If  IfExpression=u1 == 1
  If Action Subsystem : Subsystem  TreatAsAtomicUnit=on
  Manual Switch : ManualSwitch
  Merge : Merge
  Merge1 : Merge
  Merge2 : Merge
  Subsystem : Subsystem
  logic based : Constant
  time Vs carrier : Constant  Value=0
  S1 : Outport
  S3 : Outport  Port=2
  S5 : Outport  Port=3
  wires:
  T1/1 -> If Action Subsystem/1(T1), Subsystem/1(T1)
  T2/1 -> If Action Subsystem/2(T2), Subsystem/2(T2)
  T0/1 -> If Action Subsystem/3(T0), Subsystem/3(T0)
  sec/1 -> If Action Subsystem/4(sec), Subsystem/4(sec)
  Merge/1 -> S1/1
  Merge1/1 -> S3/1
  Merge2/1 -> S5/1
  Manual Switch/1 -> If/1
  logic based/1 -> Manual Switch/1
  time Vs carrier/1 -> Manual Switch/2
  If/1 -> Subsystem/Action
  If/2 -> If Action Subsystem/Action
  Subsystem/1(S1) -> Merge/1
  Subsystem/2(S3) -> Merge1/1
  Subsystem/3(S5) -> Merge2/1
  If Action Subsystem/1(S1) -> Merge/2
  If Action Subsystem/2(S3) -> Merge1/2
  If Action Subsystem/3(S5) -> Merge2/2

== system HighSpeedOperation/Subsystem/Constant Torque region ==
  Action Port : ActionPort  ActionPortLabel=if(u1 < Wbase_FW_RegionI)
  Constant : Constant  Value=I_rated
  Gain : Gain  Gain=1/Lm
  Rated Flux : Constant  Value=lambda_r_rated
  Sqrt : Sqrt
  Square : Math  Operator=square
  Square1 : Math  Operator=square
  Subtract : Sum  Inputs=-+
  Ids* : Outport
  Iqs_max : Outport  Port=2
  wires:
  Rated Flux/1 -> Gain/1  "λdr*"
  Gain/1 -> Square/1, Ids*/1  "Ids"
  Square/1 -> Subtract/1
  Constant/1 -> Square1/1
  Square1/1 -> Subtract/2
  Sqrt/1 -> Iqs_max/1
  Subtract/1 -> Sqrt/1

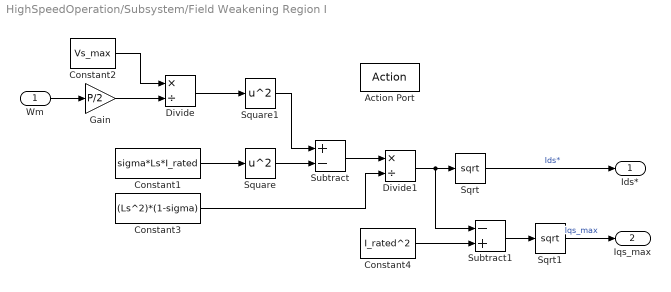
== system HighSpeedOperation/Subsystem/Field Weakening Region I ==
  Wm : Inport
  Action Port : ActionPort  ActionPortLabel=elseif(Wbase_FW_RegionI < u1 < W_BT_RegionII)
  Constant1 : Constant  Value=sigma*Ls*I_rated
  Constant2 : Constant  Value=Vs_max
  Constant3 : Constant  Value=(Ls^2)*(1-sigma)
  Constant4 : Constant  Value=I_rated^2
  Divide : Product  Inputs=*/
  Divide1 : Product  Inputs=*/
  Gain : Gain  Gain=P/2
  Sqrt : Sqrt
  Sqrt1 : Sqrt
  Square : Math  Operator=square
  Square1 : Math  Operator=square
  Subtract : Sum  Inputs=+-
  Subtract1 : Sum  Inputs=-+
  Ids* : Outport
  Iqs_max : Outport  Port=2
  wires:
  Sqrt/1 -> Ids*/1  "Ids*"
  Divide/1 -> Square1/1
  Constant1/1 -> Square/1
  Square/1 -> Subtract/2
  Square1/1 -> Subtract/1
  Constant2/1 -> Divide/1
  Wm/1 -> Gain/1
  Gain/1 -> Divide/2
  Subtract/1 -> Divide1/1
  Divide1/1 -> Subtract1/1, Sqrt/1
  Constant3/1 -> Divide1/2
  Sqrt1/1 -> Iqs_max/1  "Iqs_max"
  Constant4/1 -> Subtract1/2
  Subtract1/1 -> Sqrt1/1

== system HighSpeedOperation/Subsystem/Field Weakening Region II ==
  Wm : Inport
  Action Port : ActionPort  ActionPortLabel=else
  Constant : Constant  Value=Vs_max
  Constant1 : Constant  Value=sigma
  Divide : Product  Inputs=*/
  Divide1 : Product  Inputs=*/
  Gain : Gain  Gain=Ls*sqrt(2)
  Gain1 : Gain  Gain=P/2
  Ids* : Outport
  Iqs_max : Outport  Port=2
  wires:
  Divide1/1 -> Iqs_max/1
  Divide/1 -> Divide1/1, Ids*/1
  Constant/1 -> Divide/1
  Gain/1 -> Divide/2
  Gain1/1 -> Gain/1
  Wm/1 -> Gain1/1
  Constant1/1 -> Divide1/2
